simulink library "QuaternionLibrary"  (R2015b)
settings: Solver=VariableStepAuto  StartTime=0.0  StopTime=10.0  RelTol=1e-3
settings Model: Creator=jeremie  LastModifiedBy=jeremie

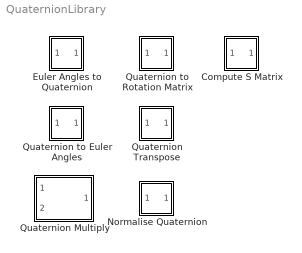
== system QuaternionLibrary ==
  Compute S Matrix : Subsystem
      mask help: Convert an orientation quaternion to an orthogonal transformation matrix
      mask Help:
      | Convert a quaternion
      | [q1 q2 q3 q4]
      | to the S matrix used to compute angular acceleration and velocity quaternion
      | qDot = S * nuBody
      | 
      | qDDot = SDot * nuBody + S * nuBodyDot
      mask Display: disp('S')
  Euler Angles to Quaternion : Subsystem
      mask help: Convert vector of Euler angles to an orientation quaternion
      mask Help:
      | Convert vector of Euler angles
      | [roll, pitch, yaw]
      | to an orientation quaternion
      | [q1 q2 q3 q4]
      | where:
      | - q1 is the rotation in radians
      | - [q2 q3 q4] is the vector around which the rotation is performed)
      | 
      | Based on code from the PX4 firmware: https://github.com/PX4/Firmware
      mask Display: disp('E2Q')
  Normalise Quaternion : Subsystem
      mask help:
      | Normalise a quaternion
      |
      | Qhat = Q / |Q|
      mask Display: disp('Q/|Q|')
  Quaternion Transpose : Subsystem
      mask help:
      | Find the transpose Q* of a quaternion Q
      |
      | [Q1* Q2* Q3* Q4*] = [Q1 -Q2 -Q3 -Q4]
      mask Display: disp('Q*')
  Quaternion to Euler Angles : Subsystem
      mask help: Convert an orientation quaternion to a vector of Euler angles
      mask Help:
      | Convert an orientation quaternion
      | [q1 q2 q3 q4]
      | where:
      | - q1 is the rotation in radians
      | - [q2 q3 q4] is the vector around which the rotation is performed)
      | to a vector of Euler angles
      | [roll, pitch, yaw]
      | Based on code from the PX4 firmware: https://github.com/PX4/Firmware
      mask Display: disp('Q2E')
  Quaternion to Rotation Matrix : Subsystem
      mask help: Convert an orientation quaternion to an orthogonal transformation matrix
      mask Help:
      | Convert an orientation quaternion
      | [q1 q2 q3 q4]
      | where:
      | - q1 is the rotation in radians
      | - [q2 q3 q4] is the vector around which the rotation is performed)
      | to an orthogonal transformation matrix
      | Based on code from the PX4 firmware: https://github.com/PX4/Firmware
      mask Display: disp('Q2R')
  Quaternion Multiply : Subsystem
      mask help:
      | Multiply two quaternions together
      |
      | Output = input1 (top) * input2 (bottom)
      mask Display: disp('Quaternion\nMultiply')

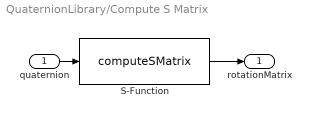
== system QuaternionLibrary/Compute S Matrix ==
  quaternion : Inport
  S-Function : S-Function  FunctionName=computeSMatrix  SFunctionDeploymentMode=off  EnableBusSupport=off
  rotationMatrix : Outport
  wires:
  S-Function/1 -> rotationMatrix/1
  quaternion/1 -> S-Function/1

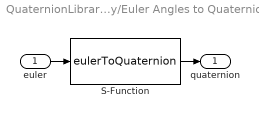
== system QuaternionLibrary/Euler Angles to Quaternion ==
  euler : Inport
  S-Function : S-Function  FunctionName=eulerToQuaternion  SFunctionDeploymentMode=off  EnableBusSupport=off
  quaternion : Outport
  wires:
  euler/1 -> S-Function/1
  S-Function/1 -> quaternion/1

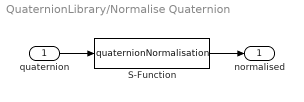
== system QuaternionLibrary/Normalise Quaternion ==
  quaternion : Inport
  S-Function : S-Function  FunctionName=quaternionNormalisation  SFunctionDeploymentMode=off  EnableBusSupport=off
  normalised : Outport
  wires:
  S-Function/1 -> normalised/1
  quaternion/1 -> S-Function/1

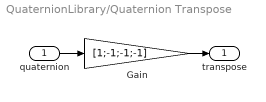
== system QuaternionLibrary/Quaternion Transpose ==
  quaternion : Inport
  Gain : Gain  Gain=[1;-1;-1;-1]
  transpose : Outport
  wires:
  quaternion/1 -> Gain/1
  Gain/1 -> transpose/1

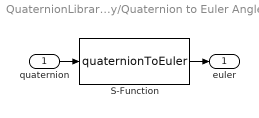
== system QuaternionLibrary/Quaternion to Euler Angles ==
  quaternion : Inport
  S-Function : S-Function  FunctionName=quaternionToEuler  SFunctionDeploymentMode=off  EnableBusSupport=off
  euler : Outport
  wires:
  S-Function/1 -> euler/1
  quaternion/1 -> S-Function/1

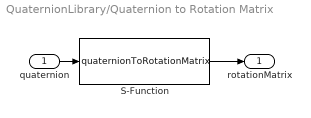
== system QuaternionLibrary/Quaternion to Rotation Matrix ==
  quaternion : Inport
  S-Function : S-Function  FunctionName=quaternionToRotationMatrix  SFunctionDeploymentMode=off  EnableBusSupport=off
  rotationMatrix : Outport
  wires:
  quaternion/1 -> S-Function/1
  S-Function/1 -> rotationMatrix/1

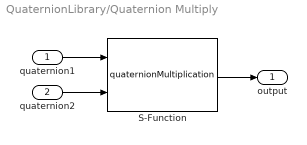
== system QuaternionLibrary/Quaternion Multiply ==
  quaternion1 : Inport
  quaternion2 : Inport  Port=2
  S-Function : S-Function  FunctionName=quaternionMultiplication  SFunctionDeploymentMode=off  EnableBusSupport=off
  output : Outport
  wires:
  quaternion1/1 -> S-Function/1
  S-Function/1 -> output/1
  quaternion2/1 -> S-Function/2
